simulink model "foc_7"  (R2024a)
settings: Solver=FixedStepAuto  StartTime=0.0  StopTime=3  FixedStep=1e-6  MaxStep=1e-5  RelTol=1e-3
undefined symbols (not defined in the file): DiscIntNeverNeededParam, Ki, Ki_s, Kp, Kp_s, L, lambda, ma, p, R, T_period, Vdc
libraries: simulink x13, spsIGBTDiodeLib x6, spsSeriesRLCBranchLib x6, eeGeneralControl x6, spsCurrentMeasurementLib x3, spsPermanentMagnetSynchronousMachineLib x2, spsDCVoltageSourceLib x1, spsStairGeneratorLib x1, spspowerguiLib x1
(part 1 of 2)
settings Model: Creator=Abdo  LastModifiedBy=kareem
settings SolverCC: ZeroCrossAlgorithm=Adaptive  AlgebraicLoopSolver=TrustRegion
settings OptimizationCC: DefaultParameterBehavior=Inlined  EnhancedBackFolding=on  PassReuseOutputArgsAs=Individual arguments  ZeroExternalMemoryAtStartup=off  ZeroInternalMemoryAtStartup=off  OptimizeBlockOrder=speed  DifferentSizesBufferReuse=on  OptimizationCustomize=off  EfficientTunableParamExpr=on
settings DebuggingCC: IgnoredZcDiagnostic=none  ParameterTunabilityLossMsg=error  ArithmeticOperatorsInVariantConditions=warning
settings HardwareCC: ProdBitPerChar=16  ProdBitPerInt=16  ProdBitPerPointer=32  ProdBitPerSizeT=32  ProdBitPerPtrDiffT=32  ProdLargestAtomicInteger=Integer  ProdLargestAtomicFloat=None  ProdWordSize=16  ProdHWDeviceType=Texas Instruments->C2000
settings SFSimCC: MATLABDynamicMemAlloc=off  CustomCodeUndefinedFunction=UseInterfaceOnly
settings RTWCC: Description=Embedded Coder  SystemTargetFile=ert.tlc  TemplateMakefile=ert_default_tmf  PortableWordSizes=on  GPUComputeCapability=3.5
settings CodeAppCC: ForceParamTrailComments=on  IgnoreCustomStorageClasses=off  OperatorAnnotations=on  SimulinkDataObjDesc=on  SFDataObjDesc=on  InsertBlockDesc=on
settings ERTTargetCC: TargetLangStandard=C99 (ISO)  GenerateSampleERTMain=on  InlinedParameterPlacement=NonHierarchical  ERTCustomFileTemplate=example_file_process.tlc

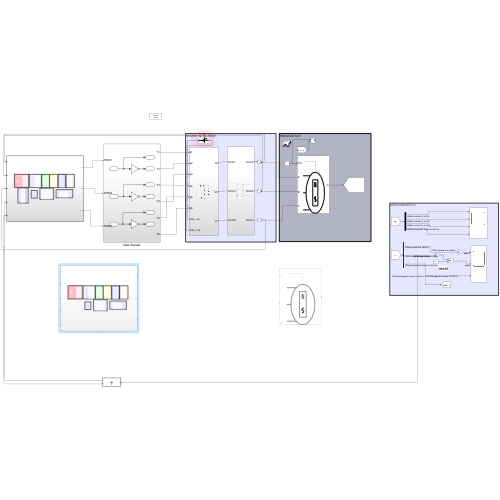
[thumbnail: Simulink's stored preview of the top-level diagram]
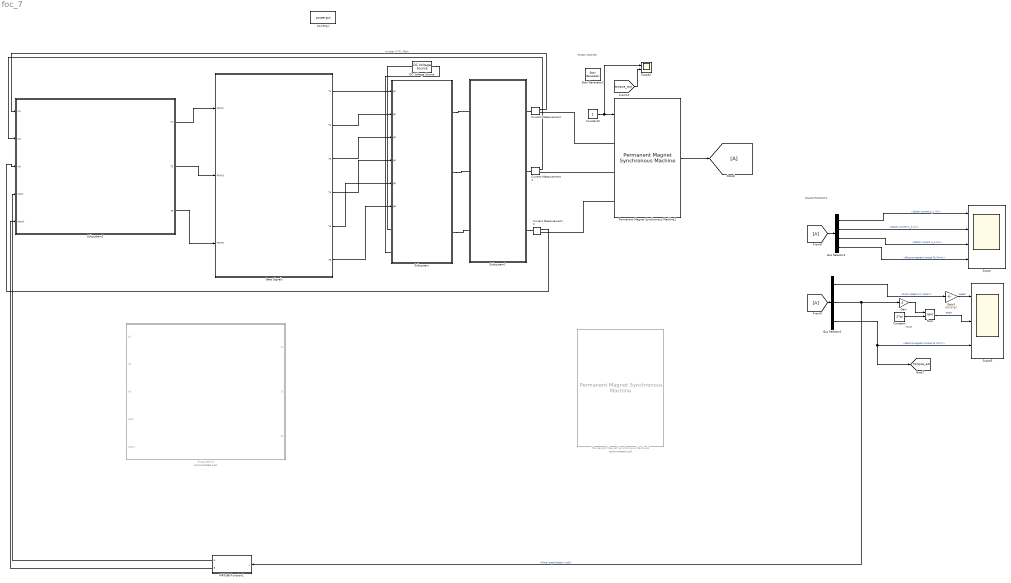
== system foc_7 ==
  note: MEASUREMENTS
  note: PMSM MOTOR
  note: inveter & RL filter
  note: reset
  Bus Selector1 : BusSelector  OutputSignals=Stator current is_c (A),Stator current is_b (A),Stator current is_a (A),Electromagnetic torque Te (N*m)
  Bus Selector2 : BusSelector  OutputSignals=Rotor speed wm (rad/s),Rotor angle thetam (rad),Electromagnetic torque Te (N*m)
  Constant : Constant  Value=2*pi
  Constant3 : Constant
  Current Measurement : spsCurrentMeasurementLib/Current Measurement  PhasorSimulation=off  OutputType=Complex  PSBequivalent=0
  Current Measurement1 : spsCurrentMeasurementLib/Current Measurement  PhasorSimulation=off  OutputType=Complex  PSBequivalent=0
  Current Measurement2 : spsCurrentMeasurementLib/Current Measurement  PhasorSimulation=off  OutputType=Complex  PSBequivalent=0
  DC Voltage Source : spsDCVoltageSourceLib/DC Voltage Source  Amplitude=Vdc  Measurements=None
  From8 : From
  From9 : From
  Gain : Gain  Gain=4
  Gain3 : Gain  Gain=60/(2*pi)
  Gate Signals : Subsystem
  Goto8 : Goto
  MATLAB Function1 : MATLAB Function  TreatAsAtomicUnit=on
  Permanent Magnet Synchronous Machine1 : spsPermanentMagnetSynchronousMachineLib/Permanent Magnet Synchronous Machine  NbPhases=3  FluxDistribution=Sinusoidal  RotorType=Round  MechanicalLoad=Torque Tm  PresetModel=No  ShowDetailedParameters=on  MeasurementBus=off  Resistance=2.9  Inductance=8.5e-3  dqInductances=[8.5e-3,8.5e-3]  La=0.0124  MachineConstant=Flux linkage established by magnets (V.s)  Flux=0.37/3  VoltageCst=89.4808  TorqueCst=0.74  Flat=120  Mechanical=[0.000026 0.000955 4 0.03]  PolePairs=4  InitialConditions=[0,0, 0,0]  InitialConditions5ph=[0 0 0 0 0 0]  RefAngle=Aligned with phase A axis (original Park)  IterativeDiscreteModel=Backward Euler robust  TsBlock=-1  TsPowergui=0
  Permanent Magnet Synchronous Machine3 : spsPermanentMagnetSynchronousMachineLib/Permanent Magnet Synchronous Machine  Commented=on  NbPhases=3  FluxDistribution=Sinusoidal  RotorType=Round  MechanicalLoad=Torque Tm  PresetModel=No  ShowDetailedParameters=on  MeasurementBus=off  Resistance=R  Inductance=8.5e-3  dqInductances=[8.5e-3,8.5e-3]  La=L  MachineConstant=Flux linkage established by magnets (V.s)  Flux=lambda  VoltageCst=62.5906  TorqueCst=0.51762  Flat=120  Mechanical=[0.000026 0.000955 4 0.03]  PolePairs=8  InitialConditions=[0 0 0 0]  InitialConditions5ph=[0 0 0 0 0 0]  RefAngle=Aligned with phase A axis (original Park)  IterativeDiscreteModel=Backward Euler robust  TsBlock=-1  TsPowergui=0
  Rem : Math  Operator=rem  SignedPower=on
  Scope : Scope  NumInputPorts=4
  Scope2 : Scope  NumInputPorts=2
  Scope5 : Scope  NumInputPorts=3
  Stair Generator2 : spsStairGeneratorLib/Stair Generator  t=[0 0.15 0.3 0.5 0.75 1 2 2.5]  e=[0 0.5 1 2 2.7 0.5 4 6]  Ts=0
  Subsystem : Subsystem
  Subsystem1 : Subsystem
  Subsystem2 : Subsystem  TreatAsAtomicUnit=on
  Subsystem3 : Subsystem  Commented=on  TreatAsAtomicUnit=on
  powergui : spspowerguiLib/powergui  Priority=1  SimulationMode=Discrete  SampleTime=1e-6  frequency=60  Iterations=50  frequencyindice=0  Pbase=100e6  ErrMax=1e-4  UnitsV=kV  UnitsW=MW  buscounter=0  FunctionMessages=off  echomessages=off  EnableUseOfTLC=off  CurrentSourceSwitches=off  DisableSnubberDevices=off  DisableRonSwitches=off  DisableVfSwitches=off  DisplayEquations=off  AutomaticDiscreteSolvers=off  SolverType=Tustin/Backward Euler (TBE)  Interpol=off  ExternalGateDelay=off  methode=off  Ts=100  x0status=blocks  SPID=on  SwTol=0  HookPort=off  NonlinearTolerance=1e-4  nMaxIteration=100  ContinueOnMaxIteration=off  RestoreLinks=warning  ResistiveCurrentMeasurement=off  Frange=[0:2:500]  Ylog=off  Xlog=on  ShowGrid=off  save=off  variable=ZData  structure=0  ZoomFFT=off  StartTime=0.0  cycles=1  DisplayStyle=1  fundamental=60  FreqAxis=off  MaxFrequency=1000  frequencyindicesteady=1  RmsSteady=1  display=off
  tag scope: torque_act=global
  wires:
  Gain/1 -> Rem/1
  Current Measurement2/1 -> Subsystem2/3(In3)
  Current Measurement1/1 -> Subsystem2/2(In2)
  Current Measurement/1 -> Subsystem2/1(In1)
  Bus Selector2/2 -> MATLAB Function1/1(u), Gain/1  "<Rotor angle thetam (rad)>"
  Constant/1 -> Rem/2
  Rem/1 -> Scope5/2  "angle"
  Permanent Magnet Synchronous Machine1/1 -> Goto8/1
  Bus Selector2/1 -> Gain3/1  "<Rotor speed wm (rad/s)>"
  Bus Selector1/1 -> Scope/1  "<Stator current is_c (A)>"
  Bus Selector1/2 -> Scope/2  "<Stator current is_b (A)>"
  Bus Selector1/3 -> Scope/3  "<Stator current is_a (A)>"
  Bus Selector1/4 -> Scope/4  "<Electromagnetic torque Te (N*m)>"
  Gain3/1 -> Scope5/1  "speed"
  Bus Selector2/3 -> [torque_act], Scope5/3  "<Electromagnetic torque Te (N*m)>"
  From8/1 -> Bus Selector1/1
  From9/1 -> Bus Selector2/1
  Constant3/1 -> Permanent Magnet Synchronous Machine1/1, Scope2/1
  [torque_act] -> Scope2/2
  MATLAB Function1/1(A) -> Subsystem2/4(Input)
  MATLAB Function1/2(B) -> Subsystem2/5(Input1)
  Gate Signals/1(T1) -> Subsystem/1(g1)
  Gate Signals/2(T2) -> Subsystem/2(g2)
  Gate Signals/3(T3) -> Subsystem/3(g3)
  Gate Signals/4(T4) -> Subsystem/4(g4)
  Gate Signals/5(T5) -> Subsystem/5(g5)
  Gate Signals/6(T6) -> Subsystem/6(g6)
  Subsystem2/1(T1) -> Gate Signals/1(PWM1)
  Subsystem2/2(T3) -> Gate Signals/2(PWM3)
  Subsystem2/3(T5) -> Gate Signals/3(PWM5)
  connections:
  Permanent Magnet Synchronous Machine1/LConn1 -- Current Measurement/RConn1
  Subsystem/LConn1 -- DC Voltage Source/LConn1
  Permanent Magnet Synchronous Machine1/LConn2 -- Current Measurement1/RConn1
  DC Voltage Source/RConn1 -- Subsystem/LConn2
  Permanent Magnet Synchronous Machine1/LConn3 -- Current Measurement2/RConn1
  Subsystem/RConn1 -- Subsystem1/LConn1
  Subsystem1/RConn1 -- Current Measurement/LConn1
  Subsystem/RConn2 -- Subsystem1/LConn2
  Subsystem1/RConn2 -- Current Measurement1/LConn1
  Subsystem1/RConn3 -- Current Measurement2/LConn1
  Subsystem/RConn3 -- Subsystem1/LConn3

== system foc_7/Gate Signals ==
  PWM1 : Inport
  PWM3 : Inport  Port=2
  PWM5 : Inport  Port=3
  NOT : Logic  Operator=NOT  IconShape=distinctive  AllPortsSameDT=off  OutDataTypeStr=boolean
  NOT1 : Logic  Operator=NOT  IconShape=distinctive  AllPortsSameDT=off  OutDataTypeStr=boolean
  NOT2 : Logic  Operator=NOT  IconShape=distinctive  AllPortsSameDT=off  OutDataTypeStr=boolean
  T1 : Outport
  T2 : Outport  Port=2
  T3 : Outport  Port=3
  T4 : Outport  Port=4
  T5 : Outport  Port=5
  T6 : Outport  Port=6
  wires:
  PWM1/1 -> T1/1, NOT/1
  NOT/1 -> T4/1
  NOT1/1 -> T6/1
  PWM3/1 -> T3/1, NOT1/1
  PWM5/1 -> T5/1, NOT2/1
  NOT2/1 -> T2/1

== system foc_7/Subsystem ==
  g1 : Inport
  g2 : Inport  Port=2
  g3 : Inport  Port=3
  g4 : Inport  Port=4
  g5 : Inport  Port=5
  g6 : Inport  Port=6
  IGBT/Diode{,1..5} (6 alike) : spsIGBTDiodeLib/IGBT//Diode  Ron=1e-3  Rs=1e5  Cs=inf  Measurements=off
  Vdc_-ve : PMIOPort  Side=Left
  Vdc_+ve : PMIOPort  Port=2  Side=Left
  Va : PMIOPort  Port=3  Side=Right
  Vb : PMIOPort  Port=4  Side=Right
  Vc : PMIOPort  Port=5  Side=Right
  wires:
  g2/1 -> IGBT/Diode5/1
  g5/1 -> IGBT/Diode4/1
  g3/1 -> IGBT/Diode2/1
  g4/1 -> IGBT/Diode1/1
  g1/1 -> IGBT/Diode/1
  g6/1 -> IGBT/Diode3/1
  connections:
  IGBT/Diode5/LConn1 -- Vc/RConn1 -- IGBT/Diode4/RConn1
  Vb/RConn1 -- IGBT/Diode3/LConn1 -- IGBT/Diode2/RConn1
  IGBT/Diode5/RConn1 -- Vdc_-ve/RConn1 -- IGBT/Diode1/RConn1 -- IGBT/Diode3/RConn1
  IGBT/Diode4/LConn1 -- IGBT/Diode/LConn1 -- Vdc_+ve/RConn1 -- IGBT/Diode2/LConn1
  Va/RConn1 -- IGBT/Diode/RConn1 -- IGBT/Diode1/LConn1

== system foc_7/Subsystem1 ==
  Series RLC Branch10 : spsSeriesRLCBranchLib/Series RLC Branch  LConnTagsString=__new0  RConnTagsString=__new0  BranchType=R  Resistance=10e4  Inductance=1e-2  SetiL0=off  InitialCurrent=0  Capacitance=1e-6  Setx0=off  InitialVoltage=0  Measurements=None
  Series RLC Branch11 : spsSeriesRLCBranchLib/Series RLC Branch  LConnTagsString=__new0  RConnTagsString=__new0  BranchType=R  Resistance=10e4  Inductance=1e-2  SetiL0=off  InitialCurrent=0  Capacitance=1e-6  Setx0=off  InitialVoltage=0  Measurements=None
  Series RLC Branch6 : spsSeriesRLCBranchLib/Series RLC Branch  LConnTagsString=__new0  RConnTagsString=__new0  BranchType=L  Resistance=1  Inductance=4e-3  SetiL0=on  InitialCurrent=0  Capacitance=1e-6  Setx0=off  InitialVoltage=0  Measurements=None
  Series RLC Branch7 : spsSeriesRLCBranchLib/Series RLC Branch  LConnTagsString=__new0  RConnTagsString=__new0  BranchType=L  Resistance=1  Inductance=4e-3  SetiL0=on  InitialCurrent=0  Capacitance=1e-6  Setx0=off  InitialVoltage=0  Measurements=None
  Series RLC Branch8 : spsSeriesRLCBranchLib/Series RLC Branch  LConnTagsString=__new0  RConnTagsString=__new0  BranchType=L  Resistance=1  Inductance=4e-3  SetiL0=on  InitialCurrent=0  Capacitance=1e-6  Setx0=off  InitialVoltage=0  Measurements=None
  Series RLC Branch9 : spsSeriesRLCBranchLib/Series RLC Branch  LConnTagsString=__new0  RConnTagsString=__new0  BranchType=R  Resistance=10e4  Inductance=1e-2  SetiL0=off  InitialCurrent=0  Capacitance=1e-6  Setx0=off  InitialVoltage=0  Measurements=None
  Conn1 : PMIOPort  Side=Left
  Conn2 : PMIOPort  Port=2  Side=Right
  Conn3 : PMIOPort  Port=3  Side=Left
  Conn4 : PMIOPort  Port=4  Side=Right
  Conn5 : PMIOPort  Port=5  Side=Right
  Conn6 : PMIOPort  Port=6  Side=Left
  connections:
  Series RLC Branch8/LConn1 -- Series RLC Branch9/LConn1 -- Conn6/RConn1
  Series RLC Branch7/LConn1 -- Conn3/RConn1 -- Series RLC Branch10/LConn1
  Series RLC Branch7/RConn1 -- Conn4/RConn1 -- Series RLC Branch10/RConn1
  Series RLC Branch6/LConn1 -- Conn1/RConn1 -- Series RLC Branch11/LConn1
  Series RLC Branch6/RConn1 -- Conn2/RConn1 -- Series RLC Branch11/RConn1
  Series RLC Branch8/RConn1 -- Conn5/RConn1 -- Series RLC Branch9/RConn1

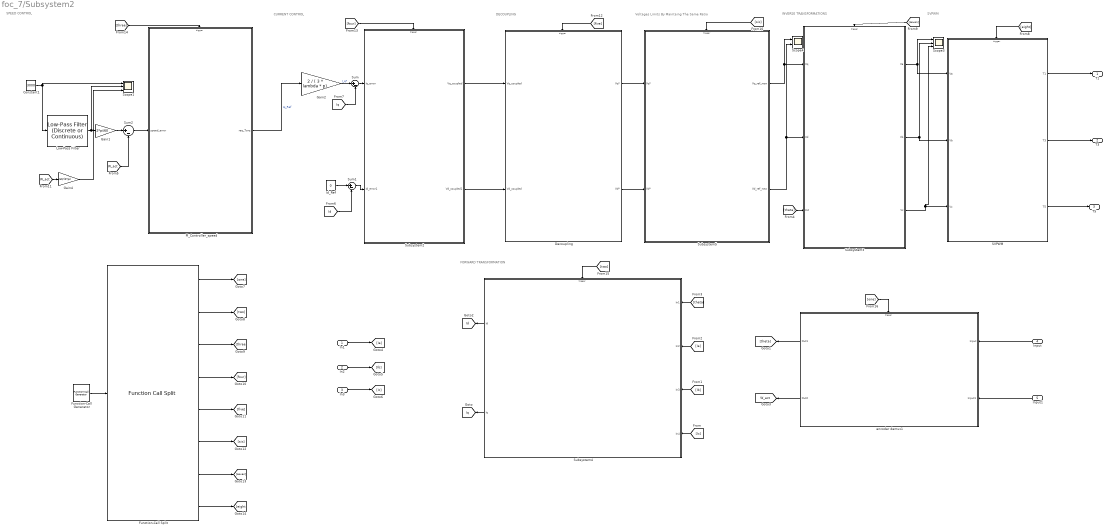
== system foc_7/Subsystem2 ==
  note: Voltages Limits By Maintaing The Same Ratio
  note: FORWARD TRANSFORMATION
  note: SPEED CONTROL
  note: CURRENT CONTROL
  note: DECOUPLING
  note: INVERSE TRANSFORMATIONS
  note: SVPWM
  In1 : Inport
  In2 : Inport  Port=2
  In3 : Inport  Port=3
  Input : Inport  Port=4
  Input1 : Inport  Port=5
  Constant1 : Constant  Value=3000
  Decoupling : Subsystem
  Function-Call Generator : simulink/Ports & Subsystems/Function-Call Generator  sample_time=1  numberOfIterations=1  DisallowWideOutput=off
  Function-Call Split : FunctionCallSplit  IconShape=distinctive  NumOutputPorts=8  OutputPortLayout=default
  Gain1 : Gain  Gain=2*pi/60
  Gain2 : Gain  Gain=2 / ( 3 * lambda * p)
  Gain4 : Gain  Gain=60/(2*pi)
  Id_Ref : Constant  Value=0
  "Low-Pass Filter " : eeGeneralControl/Low-Pass Filter (Discrete or Continuous)  K=1  T=1/100  B=inf  A=-inf  init_option=Inherited from block input  x0=0  Ts=-1
  PI_Controller_speed : Subsystem
  SVPWM : Subsystem
  Scope1 : Scope  NumInputPorts=3
  Scope3 : Scope  NumInputPorts=3
  Scope4 : Scope  NumInputPorts=2
  Subsystem2 : Subsystem
  Subsystem3 : Subsystem
  Subsystem4 : Subsystem
  Subsystem5 : Subsystem
  Sum : Sum  Inputs=|+-
  Sum1 : Sum  Inputs=|+-
  Sum2 : Sum  Inputs=|+-
  encoder demux1 : Subsystem
  T1 : Outport
  T3 : Outport  Port=2
  T5 : Outport  Port=3
  tag scope: Id=global, Iq=global, W_act=global
  wires:
  Gain4/1 -> Scope1/3
  Sum/1 -> Subsystem2/1(Iq_error)
  Constant1/1 -> "Low-Pass Filter "/1, Scope1/1
  Subsystem2/2(Vd_coupled1) -> Decoupling/2(Vd_coupled)
  Gain1/1 -> Sum2/1
  [Id] -> Sum1/2
  Decoupling/1(Vq*) -> Subsystem5/1(Vq*)
  Decoupling/2(Vd*) -> Subsystem5/2(Vd*)
  "Low-Pass Filter "/1 -> Scope1/2, Gain1/1
  Subsystem3/2(Vb) -> Scope3/2, SVPWM/2(Vb)
  Subsystem4/2(Iq) -> [Iq]
  Sum1/1 -> Subsystem2/2(Id_error1)
  Subsystem2/1(Vq_coupled) -> Decoupling/1(Vq_coupled)
  PI_Controller_speed/1(req_Torq) -> Gain2/1  "Iq_Ref"
  Subsystem5/2(Vd_ref_new) -> Subsystem3/2(Vd), Scope4/2
  Gain2/1 -> Sum/1  "I_q*"
  [W_act] -> Gain4/1
  Subsystem4/1(Id) -> [Id]
  Subsystem3/3(Vc) -> Scope3/3, SVPWM/3(Vc)
  Subsystem3/1(Va) -> Scope3/1, SVPWM/1(Va)
  Subsystem5/1(Vq_ref_new) -> Scope4/1, Subsystem3/1(Vq)
  Id_Ref/1 -> Sum1/1
  [Ic] -> Subsystem4/4(In4)
  [W_act] -> Sum2/2
  SVPWM/1(T1) -> T1/1
  [Iq] -> Sum/2
  Sum2/1 -> PI_Controller_speed/1(speed_error)
  [Ib] -> Subsystem4/3(In3)
  [theta] -> Subsystem4/1(In1)
  [Ia] -> Subsystem4/2(In2)
  [theta] -> Subsystem3/3(In2)
  SVPWM/3(T5) -> T5/1
  SVPWM/2(T3) -> T3/1
  Input/1 -> encoder demux1/1(Input)
  Input1/1 -> encoder demux1/2(Input1)
  encoder demux1/1(Out1) -> [theta]
  encoder demux1/2(Out2) -> [W_act]
  In1/1 -> [Ia]
  In2/1 -> [Ib]
  In3/1 -> [Ic]
  Function-Call Generator/1 -> Function-Call Split/1
  Function-Call Split/8 -> [eight]
  Function-Call Split/7 -> [seven]
  Function-Call Split/6 -> [six]
  Function-Call Split/5 -> [five]
  Function-Call Split/4 -> [four]
  Function-Call Split/3 -> [three]
  Function-Call Split/2 -> [two]
  Function-Call Split/1 -> [one]
  [one] -> encoder demux1/Trigger
  [two] -> Subsystem4/Trigger
  [three] -> PI_Controller_speed/Trigger
  [four] -> Subsystem2/Trigger
  [five] -> Decoupling/Trigger
  [eight] -> SVPWM/Trigger
  [seven] -> Subsystem3/Trigger
  [six] -> Subsystem5/Trigger

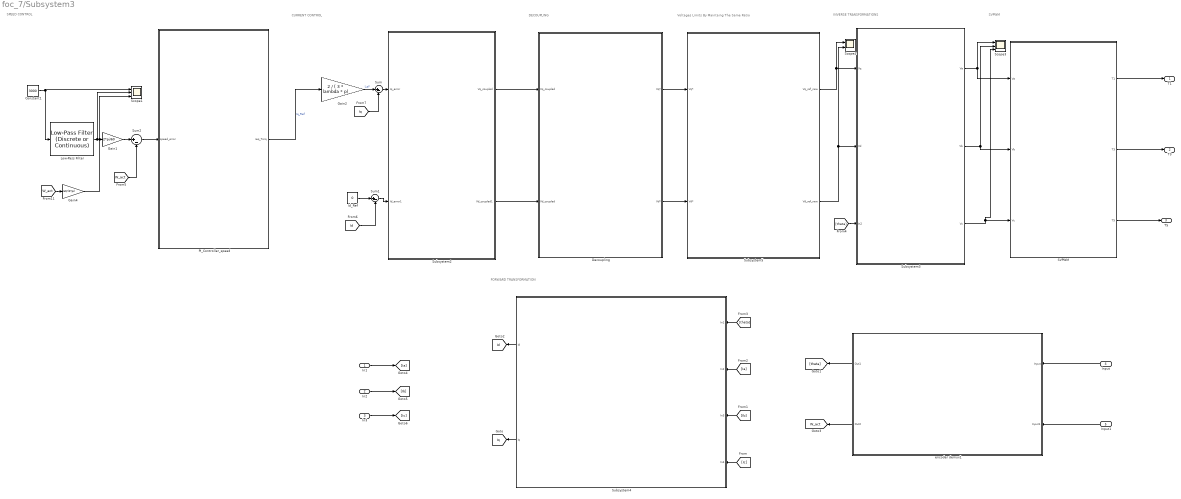
== system foc_7/Subsystem3 ==
  note: Voltages Limits By Maintaing The Same Ratio
  note: FORWARD TRANSFORMATION
  note: SPEED CONTROL
  note: CURRENT CONTROL
  note: DECOUPLING
  note: INVERSE TRANSFORMATIONS
  note: SVPWM
  In1 : Inport
  In2 : Inport  Port=2
  In3 : Inport  Port=3
  Input : Inport  Port=4
  Input1 : Inport  Port=5
  Constant1 : Constant  Value=3000
  Decoupling : Subsystem
  Gain1 : Gain  Gain=2*pi/60
  Gain2 : Gain  Gain=2 / ( 3 * lambda * p)
  Gain4 : Gain  Gain=60/(2*pi)
  Id_Ref : Constant  Value=0
  "Low-Pass Filter " : eeGeneralControl/Low-Pass Filter (Discrete or Continuous)  K=1  T=1/100  B=inf  A=-inf  init_option=Inherited from block input  x0=0  Ts=-1
  PI_Controller_speed : Subsystem
  SVPWM : Subsystem
  Scope1 : Scope  NumInputPorts=3
  Scope3 : Scope  NumInputPorts=3
  Scope4 : Scope  NumInputPorts=2
  Subsystem2 : Subsystem
  Subsystem3 : Subsystem
  Subsystem4 : Subsystem
  Subsystem5 : Subsystem
  Sum : Sum  Inputs=|+-
  Sum1 : Sum  Inputs=|+-
  Sum2 : Sum  Inputs=|+-
  encoder demux1 : Subsystem
  T1 : Outport
  T3 : Outport  Port=2
  T5 : Outport  Port=3
  tag scope: Id=global, Iq=global, W_act=global
  wires:
  Gain4/1 -> Scope1/3
  Sum/1 -> Subsystem2/1(Iq_error)
  Constant1/1 -> "Low-Pass Filter "/1, Scope1/1
  Subsystem2/2(Vd_coupled1) -> Decoupling/2(Vd_coupled)
  Gain1/1 -> Sum2/1
  [Id] -> Sum1/2
  Decoupling/1(Vq*) -> Subsystem5/1(Vq*)
  Decoupling/2(Vd*) -> Subsystem5/2(Vd*)
  "Low-Pass Filter "/1 -> Scope1/2, Gain1/1
  Subsystem3/2(Vb) -> SVPWM/2(Vb), Scope3/2
  Subsystem4/2(Iq) -> [Iq]
  Sum1/1 -> Subsystem2/2(Id_error1)
  Subsystem2/1(Vq_coupled) -> Decoupling/1(Vq_coupled)
  PI_Controller_speed/1(req_Torq) -> Gain2/1  "Iq_Ref"
  Subsystem5/2(Vd_ref_new) -> Subsystem3/2(Vd), Scope4/2
  Gain2/1 -> Sum/1  "I_q*"
  [W_act] -> Gain4/1
  Subsystem4/1(Id) -> [Id]
  Subsystem3/3(Vc) -> Scope3/3, SVPWM/3(Vc)
  Subsystem3/1(Va) -> Scope3/1, SVPWM/1(Va)
  Subsystem5/1(Vq_ref_new) -> Scope4/1, Subsystem3/1(Vq)
  Id_Ref/1 -> Sum1/1
  [Ic] -> Subsystem4/4(In4)
  [W_act] -> Sum2/2
  SVPWM/1(T1) -> T1/1
  [Iq] -> Sum/2
  Sum2/1 -> PI_Controller_speed/1(speed_error)
  [Ib] -> Subsystem4/3(In3)
  [theta] -> Subsystem4/1(In1)
  [Ia] -> Subsystem4/2(In2)
  [theta] -> Subsystem3/3(In2)
  SVPWM/3(T5) -> T5/1
  SVPWM/2(T3) -> T3/1
  Input/1 -> encoder demux1/1(Input)
  Input1/1 -> encoder demux1/2(Input1)
  encoder demux1/1(Out1) -> [theta]
  encoder demux1/2(Out2) -> [W_act]
  In1/1 -> [Ia]
  In2/1 -> [Ib]
  In3/1 -> [Ic]

== system foc_7/Subsystem2/Decoupling ==
  Vq_coupled : Inport
  Vd_coupled : Inport  Port=2
  Trigger : TriggerPort  TriggerType=function-call  VariantControl=Variant  PortDimensions=1
  Add : Sum  Inputs=+++
  Add1 : Sum  Inputs=+-
  Constant1 : Constant  Value=lambda
  Constant2 : Constant  Value=L
  Constant3 : Constant  Value=L
  Product : Product
  Product1 : Product  Inputs=3
  Product2 : Product  Inputs=3
  Vq* : Outport
  Vd* : Outport  Port=2
  wires:
  [W_act] -> Product1/1
  Product/1 -> Add/1
  Product1/1 -> Add/2
  [W_act] -> Product2/1
  Product2/1 -> Add1/2
  Constant3/1 -> Product2/3
  Constant2/1 -> Product1/3
  Constant1/1 -> Product/2
  [Id] -> Product2/2
  [W_act] -> Product/1
  [Iq] -> Product1/2
  Vd_coupled/1 -> Add1/1
  Add1/1 -> Vd*/1  "Vd"
  Add/1 -> Vq*/1  "Vq"
  Vq_coupled/1 -> Add/3

== system foc_7/Subsystem2/PI_Controller_speed ==
  speed_error : Inport
  Trigger : TriggerPort  TriggerType=function-call  VariantControl=Variant  PortDimensions=1
  Abs : Abs  SaturateOnIntegerOverflow=off
  Add : Sum
  Add1 : Sum  Inputs=+-
  Compare To Constant1 : simulink/Logic and Bit Operations/Compare To Constant  relop=<=  const=1e-4  OutDataTypeStr=boolean
  Gain3 : Gain  Gain=Kp_s
  Gain4 : Gain  Gain=Ki_s
  Integrator (Discrete or Continuous) : eeGeneralControl/Integrator (Discrete or Continuous)  LabelModeActiveChoice=Discrete  ExternalReset=level  LimitType=Anti-windup  B=4  A=-inf  Ts=-1
  Product : Product
  Saturation : Saturate  UpperLimit=3.8  LowerLimit=-3.8
  req_Torq : Outport
  wires:
  Saturation/1 -> Add1/2, req_Torq/1
  Add/1 -> Add1/1, Saturation/1
  Gain3/1 -> Add/1
  Integrator (Discrete or Continuous)/1 -> Add/2
  Gain4/1 -> Product/1
  Add1/1 -> Abs/1
  Abs/1 -> Compare To Constant1/1
  speed_error/1 -> Gain3/1, Gain4/1
  Product/1 -> Integrator (Discrete or Continuous)/1
  Compare To Constant1/1 -> Product/2

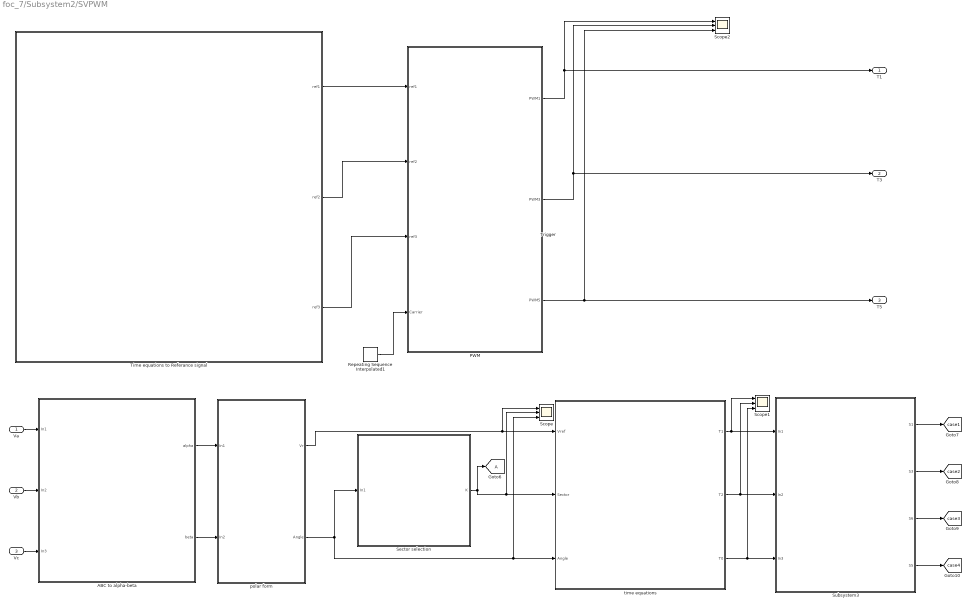
== system foc_7/Subsystem2/SVPWM ==
  Va : Inport
  Vb : Inport  Port=2
  Vc : Inport  Port=3
  Trigger : TriggerPort  TriggerType=function-call  VariantControl=Variant  PortDimensions=1
  ABC to alpha-beta : Subsystem
  Goto6 : Goto  TagVisibility=global
  PWM : Subsystem
  Repeating Sequence Interpolated1 : simulink/Sources/Repeating Sequence Interpolated  OutValues="[ 0 1/15000  1e-6  ]"  TimeValues=[ 0 1/40000 1/20001]  LookUpMeth=Interpolation-Use End Values  tsamp=1e-6  OutMin=[]  OutMax=[]  OutDataTypeStr=double  OutputDataTypeScalingMode=double  OutDataType=fixdt(0,8)  OutScaling=2^-10
  Scope : Scope  NumInputPorts=3
  Scope1 : Scope  NumInputPorts=3
  Scope2 : Scope  NumInputPorts=3
  Sector selection : Subsystem
  Subsystem3 : Subsystem
  Time equations to Referance signal : Subsystem
  polar form : Subsystem
  time equations : Subsystem
  T1 : Outport
  T3 : Outport  Port=2
  T5 : Outport  Port=3
  tag scope: case1=global, case2=global, case3=global, case4=global
  wires:
  Vb/1 -> ABC to alpha-beta/2(In2)
  time equations/1(T1) -> Scope1/1, Subsystem3/1(In1)
  Va/1 -> ABC to alpha-beta/1(In1)
  Time equations to Referance signal/1(ref1) -> PWM/1(ref1)
  Time equations to Referance signal/2("ref2 ") -> PWM/2(ref2)
  Time equations to Referance signal/3(ref3) -> PWM/3(ref3)
  Vc/1 -> ABC to alpha-beta/3(In3)
  ABC to alpha-beta/1(alpha) -> polar form/1(In1)
  ABC to alpha-beta/2(beta) -> polar form/2(In2)
  PWM/1(PWM1) -> T1/1, Scope2/1
  PWM/2(PWM3) -> T3/1, Scope2/2
  PWM/3(PWM5) -> T5/1, Scope2/3
  polar form/2(Angle) -> Sector selection/1(In1), time equations/3(Angle), Scope/3
  polar form/1(Vr) -> Scope/1, time equations/1(Vref)
  Sector selection/1(K) -> Scope/2, time equations/2(Sector), Goto6/1
  Subsystem3/2(S3) -> [case2]
  Subsystem3/1(S1) -> [case1]
  time equations/3(T0) -> Subsystem3/3(In3), Scope1/3
  time equations/2(T2) -> Scope1/2, Subsystem3/2(In2)
  Subsystem3/4(S5) -> [case4]
  Subsystem3/3(S6) -> [case3]
  Repeating Sequence Interpolated1/1 -> PWM/4(Carrier)

== system foc_7/Subsystem2/Subsystem2 ==
  Iq_error : Inport
  Id_error1 : Inport  Port=2
  Trigger : TriggerPort  TriggerType=function-call  VariantControl=Variant  PortDimensions=1
  PI_Controller_Id : Subsystem
  PI_Controller_Iq : Subsystem
  Vq_coupled : Outport
  Vd_coupled1 : Outport  Port=2
  wires:
  PI_Controller_Id/1(Vd_coupled) -> Vd_coupled1/1
  Id_error1/1 -> PI_Controller_Id/1(Id_error)
  Iq_error/1 -> PI_Controller_Iq/1(Iq_error)
  PI_Controller_Iq/1(Vq_coupled) -> Vq_coupled/1

== system foc_7/Subsystem2/Subsystem3 ==
  Vq : Inport
  Vd : Inport  Port=2
  In2 : Inport  Port=3
  Trigger : TriggerPort  TriggerType=function-call  VariantControl=Variant  PortDimensions=1
  Add : Sum
  Add1 : Sum  Inputs=-+
  Add2 : Sum  Inputs=--
  Add3 : Sum  Inputs=+-
  Cosine : Trigonometry  Operator=cos
  Cosine1 : Trigonometry
  Gain : Gain  Gain=sqrt(3)
  Gain1 : Gain  Gain=1/2
  Gain2 : Gain  Gain=1/2
  Product{,1..3} (4 alike) : Product
  Sin : Trigonometry
  Sin1 : Trigonometry  Operator=cos
  Va : Outport
  Vb : Outport  Port=2
  Vc : Outport  Port=3
  wires:
  Add/1 -> Add3/2, Add2/2, Va/1  "V_beta"
  Product2/1 -> Add1/2
  Product3/1 -> Add1/1
  Cosine/1 -> Product/1
  Sin1/1 -> Product2/1
  Sin/1 -> Product1/1
  Product/1 -> Add/2
  Vd/1 -> Product1/2, Product2/2
  In2/1 -> Sin/1, Cosine/1, Cosine1/1, Sin1/1
  Product1/1 -> Add/1
  Cosine1/1 -> Product3/2
  Add1/1 -> Gain/1  "V_alpha"
  Vq/1 -> Product3/1, Product/2
  Gain1/1 -> Vc/1  "Vc"
  Add3/1 -> Gain2/1
  Gain/1 -> Add2/1, Add3/1
  Add2/1 -> Gain1/1
  Gain2/1 -> Vb/1  "Vb"

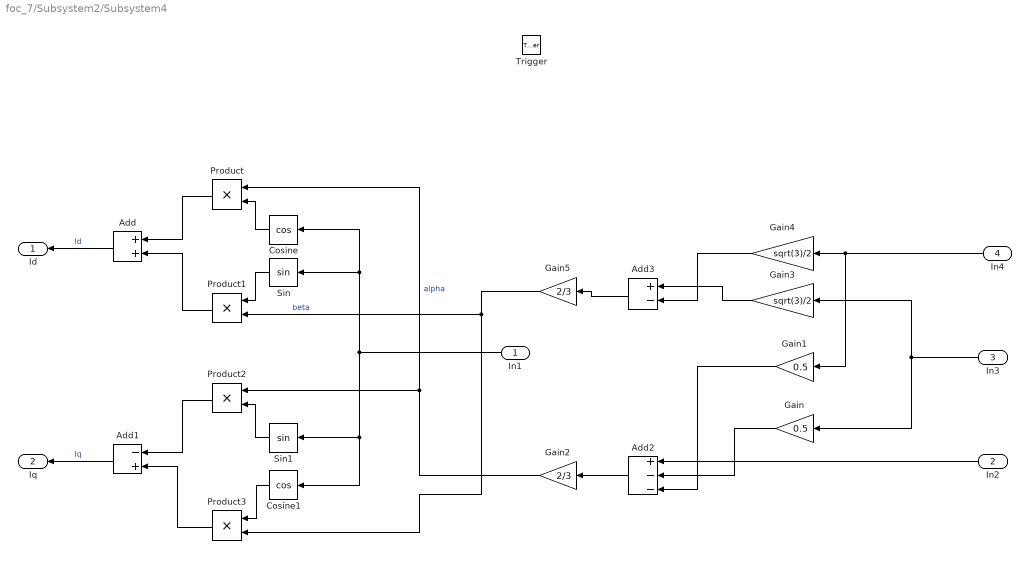
== system foc_7/Subsystem2/Subsystem4 ==
  In1 : Inport
  In2 : Inport  Port=2
  In3 : Inport  Port=3
  In4 : Inport  Port=4
  Trigger : TriggerPort  TriggerType=function-call  VariantControl=Variant  PortDimensions=1
  Add : Sum
  Add1 : Sum  Inputs=-+
  Add2 : Sum  Inputs=+--
  Add3 : Sum  Inputs=+-
  Cosine : Trigonometry  Operator=cos
  Cosine1 : Trigonometry  Operator=cos
  Gain : Gain  Gain=0.5
  Gain1 : Gain  Gain=0.5
  Gain2 : Gain  Gain=2/3
  Gain3 : Gain  Gain=sqrt(3)/2
  Gain4 : Gain  Gain=sqrt(3)/2
  Gain5 : Gain  Gain=2/3
  Product{,1..3} (4 alike) : Product
  Sin : Trigonometry
  Sin1 : Trigonometry
  Id : Outport
  Iq : Outport  Port=2
  wires:
  Add1/1 -> Iq/1  "Iq"
  Add/1 -> Id/1  "Id"
  Product3/1 -> Add1/2
  Product1/1 -> Add/2
  Sin1/1 -> Product2/2
  Sin/1 -> Product1/1
  Product/1 -> Add/1
  Cosine1/1 -> Product3/1
  In1/1 -> Cosine/1, Sin/1, Cosine1/1, Sin1/1
  Product2/1 -> Add1/1
  Cosine/1 -> Product/2
  Gain5/1 -> Product3/2, Product1/2  "beta"
  Gain2/1 -> Product/1, Product2/1  "alpha"
  Add2/1 -> Gain2/1
  In2/1 -> Add2/1
  Gain/1 -> Add2/2
  In4/1 -> Gain1/1, Gain4/1
  Gain1/1 -> Add2/3
  Add3/1 -> Gain5/1
  Gain4/1 -> Add3/2
  In3/1 -> Gain/1, Gain3/1
  Gain3/1 -> Add3/1

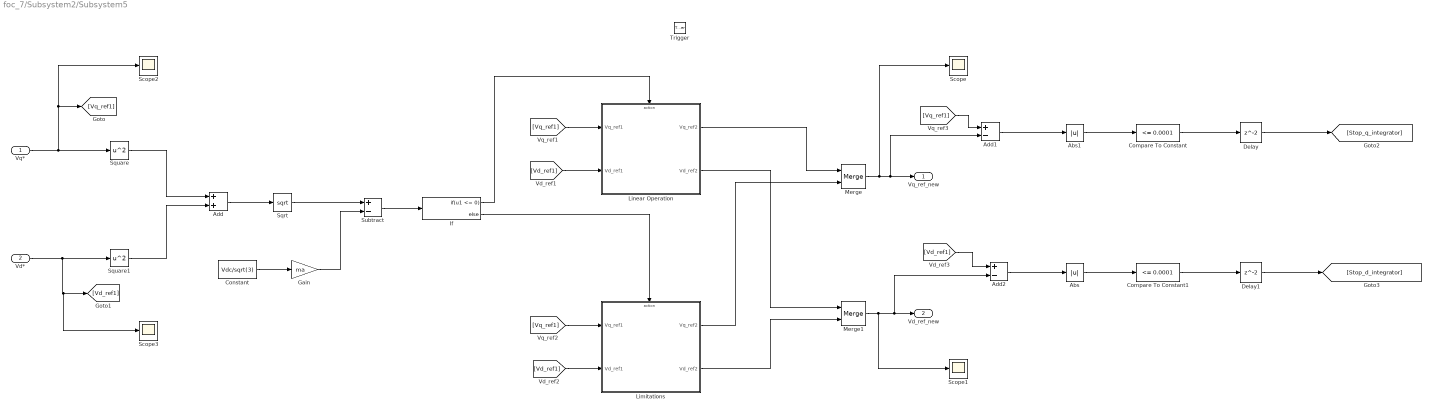
== system foc_7/Subsystem2/Subsystem5 ==
  Vq* : Inport
  Vd* : Inport  Port=2
  Trigger : TriggerPort  TriggerType=function-call  VariantControl=Variant  PortDimensions=1
  Abs : Abs  SaturateOnIntegerOverflow=off
  Abs1 : Abs  SaturateOnIntegerOverflow=off
  Add : Sum
  Add1 : Sum  Inputs=+-
  Add2 : Sum  Inputs=+-
  Compare To Constant : simulink/Logic and Bit Operations/Compare To Constant  relop=<=  const=0.0001  OutDataTypeStr=boolean
  Compare To Constant1 : simulink/Logic and Bit Operations/Compare To Constant  relop=<=  const=0.0001  OutDataTypeStr=boolean
  Constant : Constant  Value=Vdc/sqrt(3)
  Delay : Delay
  Delay1 : Delay
  Gain : Gain  Gain=ma
  If : If  IfExpression=u1 <= 0
  Limitations : Subsystem  TreatAsAtomicUnit=on
  "Linear Operation " : Subsystem  TreatAsAtomicUnit=on
  Merge : Merge
  Merge1 : Merge
  Scope{,1..3} (4 alike) : Scope
  Sqrt : Sqrt
  Square : Math  Operator=square  SignedPower=on
  Square1 : Math  Operator=square  SignedPower=on
  Subtract : Sum  Inputs=+-
  Vq_ref_new : Outport
  Vd_ref_new : Outport  Port=2
  wires:
  Vd*/1 -> Scope3/1, [Vd_ref1], Square1/1
  Vq*/1 -> Scope2/1, [Vq_ref1], Square/1
  Square/1 -> Add/1
  Square1/1 -> Add/2
  Add/1 -> Sqrt/1
  Constant/1 -> Gain/1
  Sqrt/1 -> Subtract/1
  Gain/1 -> Subtract/2
  Subtract/1 -> If/1
  [Vq_ref1] -> "Linear Operation "/1(Vq_ref1)
  [Vd_ref1] -> "Linear Operation "/2(Vd_ref1)
  If/1 -> "Linear Operation "/Action
  If/2 -> Limitations/Action
  [Vq_ref1] -> Limitations/1(Vq_ref1)
  [Vd_ref1] -> Limitations/2(Vd_ref1)
  Limitations/2(Vd_ref2) -> Merge1/2
  "Linear Operation "/2(Vd_ref2) -> Merge1/1
  Limitations/1(Vq_ref2) -> Merge/2
  "Linear Operation "/1(Vq_ref2) -> Merge/1
  Merge/1 -> Scope/1, Add1/2, Vq_ref_new/1
  Merge1/1 -> Scope1/1, Add2/2, Vd_ref_new/1
  [Vq_ref1] -> Add1/1
  [Vd_ref1] -> Add2/1
  Add2/1 -> Abs/1
  Add1/1 -> Abs1/1
  Abs1/1 -> Compare To Constant/1
  Abs/1 -> Compare To Constant1/1
  Compare To Constant/1 -> Delay/1
  Compare To Constant1/1 -> Delay1/1
  Delay/1 -> [Stop_q_integrator]
  Delay1/1 -> [Stop_d_integrator]

== system foc_7/Subsystem2/encoder demux1 ==
  Input : Inport
  Input1 : Inport  Port=2
  Trigger : TriggerPort  TriggerType=function-call  VariantControl=Variant  PortDimensions=1
  Add1 : Sum
  Constant2 : Constant
  Constant3 : Constant  Value=2*pi
  Constant4 : Constant  Value=0
  Data Type Conversion : DataTypeConversion  SaturateOnIntegerOverflow=off  RndMeth=Floor
  Data Type Conversion1 : DataTypeConversion  SaturateOnIntegerOverflow=off  RndMeth=Floor
  Detect Rise Positive : simulink/Logic and Bit Operations/Detect Rise Positive  vinit=0  OutDataTypeStr=uint8
  Discrete Derivative : simulink/Discrete/Discrete Derivative  gainval=1.0  ICPrevScaledInput=0.0  OutMin=[]  OutMax=[]  OutDataType=fixdt(1, 16)  OutScaling=2^-10  DoSatur=off
  Gain : Gain
  Gain1 : Gain  Gain=-1
  Gain2 : Gain  Gain=2*pi /2000
  Gain3 : Gain  Gain=4
  "Low-Pass Filter " : eeGeneralControl/Low-Pass Filter (Discrete or Continuous)  K=1  T=1/100  B=inf  A=-inf  init_option=Inherited from block input  x0=0  Ts=-1
  Rem : Math  Operator=rem
  Scope : Scope  NumInputPorts=3
  Switch : Switch  Criteria=u2 > Threshold  SaturateOnIntegerOverflow=off  InputSameDT=off
  Switch2 : Switch  Criteria=u2 > Threshold  SaturateOnIntegerOverflow=off  InputSameDT=off
  Unit Delay : UnitDelay  SampleTime=-1  HasFrameUpgradeWarning=on
  Out1 : Outport
  Out2 : Outport  Port=2
  wires:
  Gain3/1 -> Rem/1
  "Low-Pass Filter "/1 -> Out2/1, Scope/1
  Switch2/1 -> Switch/1
  Gain/1 -> Switch2/3
  Gain1/1 -> Switch2/1
  Data Type Conversion/1 -> Gain1/1, Gain/1
  Constant4/1 -> Switch/3
  Gain2/1 -> Gain3/1, Discrete Derivative/1, Scope/2
  Constant3/1 -> Rem/2
  Data Type Conversion1/1 -> Switch2/2
  Constant2/1 -> Data Type Conversion/1
  Switch/1 -> Add1/1, Scope/3
  Discrete Derivative/1 -> "Low-Pass Filter "/1
  Input/1 -> Detect Rise Positive/1
  Input1/1 -> Data Type Conversion1/1
  Detect Rise Positive/1 -> Switch/2
  Rem/1 -> Out1/1
  Unit Delay/1 -> Add1/2
  Add1/1 -> Gain2/1, Unit Delay/1

== system foc_7/Subsystem3/Decoupling ==
  Vq_coupled : Inport
  Vd_coupled : Inport  Port=2
  Add : Sum  Inputs=+++
  Add1 : Sum  Inputs=+-
  Constant1 : Constant  Value=lambda
  Constant2 : Constant  Value=L
  Constant3 : Constant  Value=L
  Product : Product
  Product1 : Product  Inputs=3
  Product2 : Product  Inputs=3
  Vq* : Outport
  Vd* : Outport  Port=2
  wires:
  [W_act] -> Product1/1
  Product/1 -> Add/1
  Product1/1 -> Add/2
  [W_act] -> Product2/1
  Product2/1 -> Add1/2
  Constant3/1 -> Product2/3
  Constant2/1 -> Product1/3
  Constant1/1 -> Product/2
  [Id] -> Product2/2
  [W_act] -> Product/1
  [Iq] -> Product1/2
  Vd_coupled/1 -> Add1/1
  Add1/1 -> Vd*/1  "Vd"
  Add/1 -> Vq*/1  "Vq"
  Vq_coupled/1 -> Add/3

== system foc_7/Subsystem3/PI_Controller_speed ==
  speed_error : Inport
  Abs : Abs  SaturateOnIntegerOverflow=off
  Add : Sum
  Add1 : Sum  Inputs=+-
  Compare To Constant1 : simulink/Logic and Bit Operations/Compare To Constant  relop=<=  const=1e-4  OutDataTypeStr=boolean
  Gain3 : Gain  Gain=Kp_s
  Gain4 : Gain  Gain=Ki_s
  Integrator (Discrete or Continuous) : eeGeneralControl/Integrator (Discrete or Continuous)  LabelModeActiveChoice=Discrete  ExternalReset=level  LimitType=Anti-windup  B=4  A=-inf  Ts=-1
  Product : Product
  Saturation : Saturate  UpperLimit=3.8  LowerLimit=-3.8
  req_Torq : Outport
  wires:
  Saturation/1 -> Add1/2, req_Torq/1
  Add/1 -> Add1/1, Saturation/1
  Gain3/1 -> Add/1
  Integrator (Discrete or Continuous)/1 -> Add/2
  Gain4/1 -> Product/1
  Add1/1 -> Abs/1
  Abs/1 -> Compare To Constant1/1
  speed_error/1 -> Gain3/1, Gain4/1
  Product/1 -> Integrator (Discrete or Continuous)/1
  Compare To Constant1/1 -> Product/2

== system foc_7/Subsystem3/SVPWM ==
  Va : Inport
  Vb : Inport  Port=2
  Vc : Inport  Port=3
  ABC to alpha-beta : Subsystem
  Goto6 : Goto  TagVisibility=global
  PWM : Subsystem
  Repeating Sequence Interpolated1 : simulink/Sources/Repeating Sequence Interpolated  OutValues="[ 0 1/15000  1e-6  ]"  TimeValues=[ 0 1/40000 1/20001]  LookUpMeth=Interpolation-Use End Values  tsamp=1e-6  OutMin=[]  OutMax=[]  OutDataTypeStr=double  OutputDataTypeScalingMode=double  OutDataType=fixdt(0,8)  OutScaling=2^-10
  Scope : Scope  NumInputPorts=3
  Scope1 : Scope  NumInputPorts=3
  Scope2 : Scope  NumInputPorts=3
  Sector selection : Subsystem
  Subsystem3 : Subsystem
  Time equations to Referance signal : Subsystem
  polar form : Subsystem
  time equations : Subsystem
  T1 : Outport
  T3 : Outport  Port=2
  T5 : Outport  Port=3
  tag scope: case1=global, case2=global, case3=global, case4=global
  wires:
  Vb/1 -> ABC to alpha-beta/2(In2)
  time equations/1(T1) -> Scope1/1, Subsystem3/1(In1)
  Va/1 -> ABC to alpha-beta/1(In1)
  Time equations to Referance signal/1(ref1) -> PWM/1(ref1)
  Time equations to Referance signal/2("ref2 ") -> PWM/2(ref2)
  Time equations to Referance signal/3(ref3) -> PWM/3(ref3)
  Vc/1 -> ABC to alpha-beta/3(In3)
  ABC to alpha-beta/1(alpha) -> polar form/1(In1)
  ABC to alpha-beta/2(beta) -> polar form/2(In2)
  PWM/1(PWM1) -> T1/1, Scope2/1
  PWM/2(PWM3) -> T3/1, Scope2/2
  PWM/3(PWM5) -> T5/1, Scope2/3
  polar form/2(Angle) -> Sector selection/1(In1), time equations/3(Angle), Scope/3
  polar form/1(Vr) -> Scope/1, time equations/1(Vref)
  Sector selection/1(K) -> Scope/2, time equations/2(Sector), Goto6/1
  Subsystem3/2(S3) -> [case2]
  Subsystem3/1(S1) -> [case1]
  time equations/3(T0) -> Subsystem3/3(In3), Scope1/3
  time equations/2(T2) -> Scope1/2, Subsystem3/2(In2)
  Subsystem3/4(S5) -> [case4]
  Subsystem3/3(S6) -> [case3]
  Repeating Sequence Interpolated1/1 -> PWM/4(Carrier)

== system foc_7/Subsystem3/Subsystem2 ==
  Iq_error : Inport
  Id_error1 : Inport  Port=2
  PI_Controller_Id : Subsystem
  PI_Controller_Iq : Subsystem
  Vq_coupled : Outport
  Vd_coupled1 : Outport  Port=2
  wires:
  PI_Controller_Id/1(Vd_coupled) -> Vd_coupled1/1
  Id_error1/1 -> PI_Controller_Id/1(Id_error)
  Iq_error/1 -> PI_Controller_Iq/1(Iq_error)
  PI_Controller_Iq/1(Vq_coupled) -> Vq_coupled/1

== system foc_7/Subsystem3/Subsystem3 ==
  Vq : Inport
  Vd : Inport  Port=2
  In2 : Inport  Port=3
  Add : Sum
  Add1 : Sum  Inputs=-+
  Add2 : Sum  Inputs=--
  Add3 : Sum  Inputs=+-
  Cosine : Trigonometry  Operator=cos
  Cosine1 : Trigonometry
  Gain : Gain  Gain=sqrt(3)
  Gain1 : Gain  Gain=1/2
  Gain2 : Gain  Gain=1/2
  Product{,1..3} (4 alike) : Product
  Sin : Trigonometry
  Sin1 : Trigonometry  Operator=cos
  Va : Outport
  Vb : Outport  Port=2
  Vc : Outport  Port=3
  wires:
  Add/1 -> Add3/2, Add2/2, Va/1  "V_beta"
  Product2/1 -> Add1/2
  Product3/1 -> Add1/1
  Cosine/1 -> Product/1
  Sin1/1 -> Product2/1
  Sin/1 -> Product1/1
  Product/1 -> Add/2
  Vd/1 -> Product1/2, Product2/2
  In2/1 -> Sin/1, Cosine/1, Cosine1/1, Sin1/1
  Product1/1 -> Add/1
  Cosine1/1 -> Product3/2
  Add1/1 -> Gain/1  "V_alpha"
  Vq/1 -> Product3/1, Product/2
  Gain1/1 -> Vc/1  "Vc"
  Add3/1 -> Gain2/1
  Gain/1 -> Add2/1, Add3/1
  Add2/1 -> Gain1/1
  Gain2/1 -> Vb/1  "Vb"

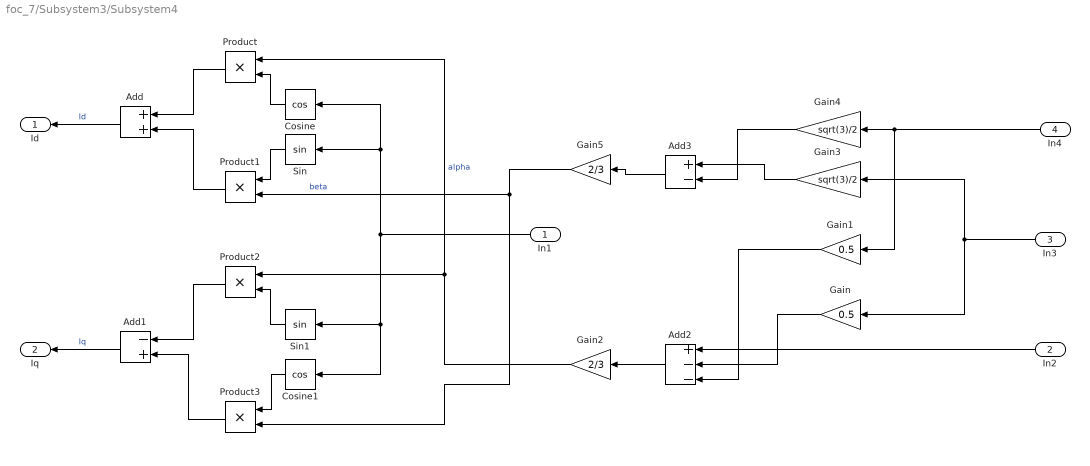
== system foc_7/Subsystem3/Subsystem4 ==
  In1 : Inport
  In2 : Inport  Port=2
  In3 : Inport  Port=3
  In4 : Inport  Port=4
  Add : Sum
  Add1 : Sum  Inputs=-+
  Add2 : Sum  Inputs=+--
  Add3 : Sum  Inputs=+-
  Cosine : Trigonometry  Operator=cos
  Cosine1 : Trigonometry  Operator=cos
  Gain : Gain  Gain=0.5
  Gain1 : Gain  Gain=0.5
  Gain2 : Gain  Gain=2/3
  Gain3 : Gain  Gain=sqrt(3)/2
  Gain4 : Gain  Gain=sqrt(3)/2
  Gain5 : Gain  Gain=2/3
  Product{,1..3} (4 alike) : Product
  Sin : Trigonometry
  Sin1 : Trigonometry
  Id : Outport
  Iq : Outport  Port=2
  wires:
  Add1/1 -> Iq/1  "Iq"
  Add/1 -> Id/1  "Id"
  Product3/1 -> Add1/2
  Product1/1 -> Add/2
  Sin1/1 -> Product2/2
  Sin/1 -> Product1/1
  Product/1 -> Add/1
  Cosine1/1 -> Product3/1
  In1/1 -> Cosine/1, Sin/1, Cosine1/1, Sin1/1
  Product2/1 -> Add1/1
  Cosine/1 -> Product/2
  Gain5/1 -> Product3/2, Product1/2  "beta"
  Gain2/1 -> Product/1, Product2/1  "alpha"
  Add2/1 -> Gain2/1
  In2/1 -> Add2/1
  Gain/1 -> Add2/2
  In4/1 -> Gain1/1, Gain4/1
  Gain1/1 -> Add2/3
  Add3/1 -> Gain5/1
  Gain4/1 -> Add3/2
  In3/1 -> Gain/1, Gain3/1
  Gain3/1 -> Add3/1

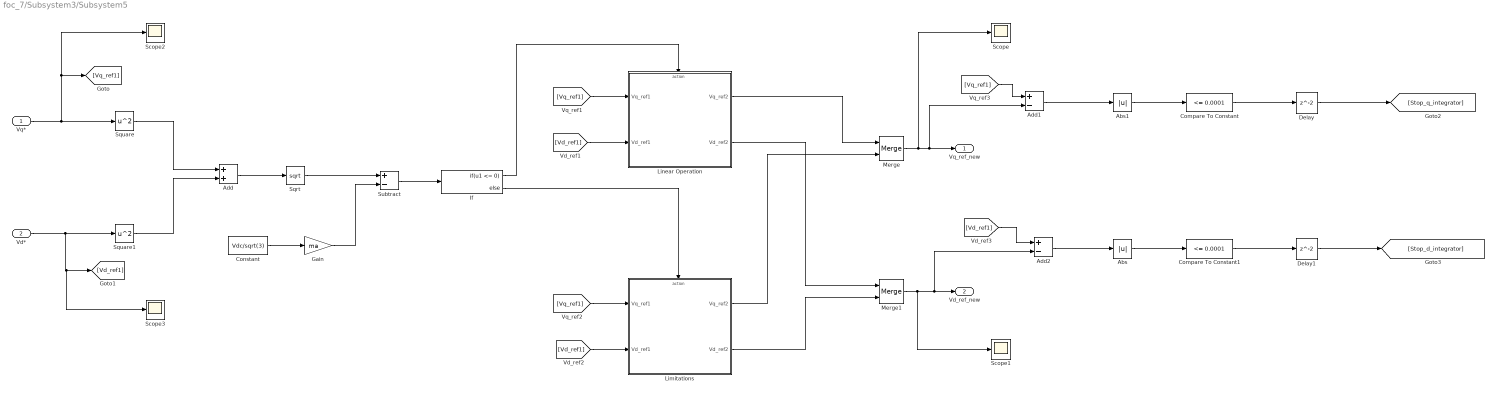
== system foc_7/Subsystem3/Subsystem5 ==
  Vq* : Inport
  Vd* : Inport  Port=2
  Abs : Abs  SaturateOnIntegerOverflow=off
  Abs1 : Abs  SaturateOnIntegerOverflow=off
  Add : Sum
  Add1 : Sum  Inputs=+-
  Add2 : Sum  Inputs=+-
  Compare To Constant : simulink/Logic and Bit Operations/Compare To Constant  relop=<=  const=0.0001  OutDataTypeStr=boolean
  Compare To Constant1 : simulink/Logic and Bit Operations/Compare To Constant  relop=<=  const=0.0001  OutDataTypeStr=boolean
  Constant : Constant  Value=Vdc/sqrt(3)
  Delay : Delay
  Delay1 : Delay
  Gain : Gain  Gain=ma
  If : If  IfExpression=u1 <= 0
  Limitations : Subsystem  TreatAsAtomicUnit=on
  "Linear Operation " : Subsystem  TreatAsAtomicUnit=on
  Merge : Merge
  Merge1 : Merge
  Scope{,1..3} (4 alike) : Scope
  Sqrt : Sqrt
  Square : Math  Operator=square  SignedPower=on
  Square1 : Math  Operator=square  SignedPower=on
  Subtract : Sum  Inputs=+-
  Vq_ref_new : Outport
  Vd_ref_new : Outport  Port=2
  wires:
  Vd*/1 -> Scope3/1, [Vd_ref1], Square1/1
  Vq*/1 -> Scope2/1, [Vq_ref1], Square/1
  Square/1 -> Add/1
  Square1/1 -> Add/2
  Add/1 -> Sqrt/1
  Constant/1 -> Gain/1
  Sqrt/1 -> Subtract/1
  Gain/1 -> Subtract/2
  Subtract/1 -> If/1
  [Vq_ref1] -> "Linear Operation "/1(Vq_ref1)
  [Vd_ref1] -> "Linear Operation "/2(Vd_ref1)
  If/1 -> "Linear Operation "/Action
  If/2 -> Limitations/Action
  [Vq_ref1] -> Limitations/1(Vq_ref1)
  [Vd_ref1] -> Limitations/2(Vd_ref1)
  Limitations/2(Vd_ref2) -> Merge1/2
  "Linear Operation "/2(Vd_ref2) -> Merge1/1
  Limitations/1(Vq_ref2) -> Merge/2
  "Linear Operation "/1(Vq_ref2) -> Merge/1
  Merge/1 -> Scope/1, Add1/2, Vq_ref_new/1
  Merge1/1 -> Scope1/1, Add2/2, Vd_ref_new/1
  [Vq_ref1] -> Add1/1
  [Vd_ref1] -> Add2/1
  Add2/1 -> Abs/1
  Add1/1 -> Abs1/1
  Abs1/1 -> Compare To Constant/1
  Abs/1 -> Compare To Constant1/1
  Compare To Constant/1 -> Delay/1
  Compare To Constant1/1 -> Delay1/1
  Delay/1 -> [Stop_q_integrator]
  Delay1/1 -> [Stop_d_integrator]

== system foc_7/Subsystem3/encoder demux1 ==
  Input : Inport
  Input1 : Inport  Port=2
  Add1 : Sum
  Constant2 : Constant
  Constant3 : Constant  Value=2*pi
  Constant4 : Constant  Value=0
  Data Type Conversion : DataTypeConversion  SaturateOnIntegerOverflow=off  RndMeth=Floor
  Data Type Conversion1 : DataTypeConversion  SaturateOnIntegerOverflow=off  RndMeth=Floor
  Detect Rise Positive : simulink/Logic and Bit Operations/Detect Rise Positive  vinit=0  OutDataTypeStr=uint8
  Discrete Derivative : simulink/Discrete/Discrete Derivative  gainval=1.0  ICPrevScaledInput=0.0  OutMin=[]  OutMax=[]  OutDataType=fixdt(1, 16)  OutScaling=2^-10  DoSatur=off
  Gain : Gain
  Gain1 : Gain  Gain=-1
  Gain2 : Gain  Gain=2*pi /2000
  Gain3 : Gain  Gain=4
  "Low-Pass Filter " : eeGeneralControl/Low-Pass Filter (Discrete or Continuous)  K=1  T=1/100  B=inf  A=-inf  init_option=Inherited from block input  x0=0  Ts=-1
  Rem : Math  Operator=rem
  Scope : Scope  NumInputPorts=3
  Switch : Switch  Criteria=u2 > Threshold  SaturateOnIntegerOverflow=off  InputSameDT=off
  Switch2 : Switch  Criteria=u2 > Threshold  SaturateOnIntegerOverflow=off  InputSameDT=off
  Unit Delay : UnitDelay  SampleTime=-1  HasFrameUpgradeWarning=on
  Out1 : Outport
  Out2 : Outport  Port=2
  wires:
  Gain3/1 -> Rem/1
  "Low-Pass Filter "/1 -> Out2/1, Scope/1
  Switch2/1 -> Switch/1
  Gain/1 -> Switch2/3
  Gain1/1 -> Switch2/1
  Data Type Conversion/1 -> Gain1/1, Gain/1
  Constant4/1 -> Switch/3
  Gain2/1 -> Gain3/1, Discrete Derivative/1, Scope/2
  Constant3/1 -> Rem/2
  Data Type Conversion1/1 -> Switch2/2
  Constant2/1 -> Data Type Conversion/1
  Switch/1 -> Add1/1, Scope/3
  Discrete Derivative/1 -> "Low-Pass Filter "/1
  Input/1 -> Detect Rise Positive/1
  Input1/1 -> Data Type Conversion1/1
  Detect Rise Positive/1 -> Switch/2
  Rem/1 -> Out1/1
  Unit Delay/1 -> Add1/2
  Add1/1 -> Gain2/1, Unit Delay/1

== system foc_7/Subsystem2/SVPWM/ABC to alpha-beta ==
  In1 : Inport
  In2 : Inport  Port=2
  In3 : Inport  Port=3
  Add : Sum  Inputs=+--
  Add1 : Sum  Inputs=+-
  Gain : Gain  Gain=0.5
  Gain1 : Gain  Gain=0.5
  Gain2 : Gain  Gain=2/3
  Gain3 : Gain  Gain=sqrt(3)/2
  Gain4 : Gain  Gain=sqrt(3)/2
  Gain5 : Gain  Gain=2/3
  Scope1 : Scope  NumInputPorts=3
  alpha : Outport
  beta : Outport  Port=2
  wires:
  Gain3/1 -> Add1/1
  In2/1 -> Gain3/1, Scope1/2, Gain/1
  Gain4/1 -> Add1/2
  Add1/1 -> Gain5/1
  Gain1/1 -> Add/3
  In3/1 -> Scope1/3, Gain4/1, Gain1/1
  Gain/1 -> Add/2
  In1/1 -> Add/1, Scope1/1
  Add/1 -> Gain2/1
  Gain2/1 -> alpha/1  "alpha"
  Gain5/1 -> beta/1  "beta"

== system foc_7/Subsystem2/SVPWM/PWM ==
  ref1 : Inport
  ref2 : Inport  Port=2
  ref3 : Inport  Port=3
  Carrier : Inport  Port=4
  Relational Operator : RelationalOperator  OutDataTypeStr=boolean  RndMeth=Simplest  InputSameDT=off
  Relational Operator1 : RelationalOperator  OutDataTypeStr=boolean  RndMeth=Simplest  InputSameDT=off
  Relational Operator2 : RelationalOperator  OutDataTypeStr=boolean  RndMeth=Simplest  InputSameDT=off
  PWM1 : Outport
  PWM3 : Outport  Port=2
  PWM5 : Outport  Port=3
  wires:
  ref1/1 -> Relational Operator/1
  ref2/1 -> Relational Operator1/1
  ref3/1 -> Relational Operator2/1
  Carrier/1 -> Relational Operator/2, Relational Operator2/2, Relational Operator1/2
  Relational Operator/1 -> PWM1/1
  Relational Operator1/1 -> PWM3/1
  Relational Operator2/1 -> PWM5/1

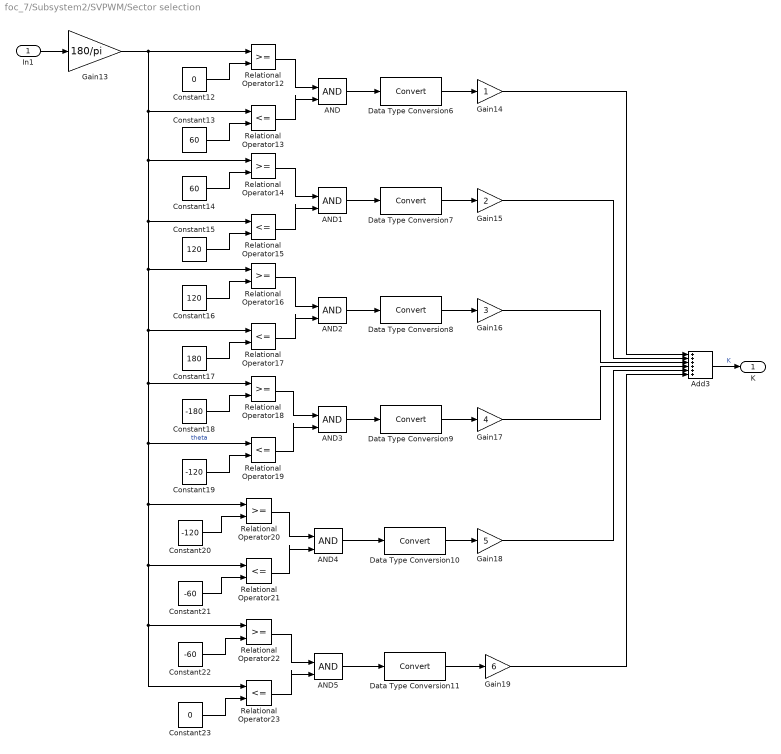
== system foc_7/Subsystem2/SVPWM/Sector selection ==
  In1 : Inport
  AND{,1..5} (6 alike) : Logic  IconShape=distinctive  AllPortsSameDT=off  OutDataTypeStr=boolean
  Add3 : Sum  Inputs=++++++
  Constant12 : Constant  Value=0
  Constant13 : Constant  Value=60
  Constant14 : Constant  Value=60
  Constant15 : Constant  Value=120
  Constant16 : Constant  Value=120
  Constant17 : Constant  Value=180
  Constant18 : Constant  Value=-180
  Constant19 : Constant  Value=-120
  Constant20 : Constant  Value=-120
  Constant21 : Constant  Value=-60
  Constant22 : Constant  Value=-60
  Constant23 : Constant  Value=0
  Data Type Conversion{6..11} (6 alike) : DataTypeConversion  SaturateOnIntegerOverflow=off  RndMeth=Floor
  Gain13 : Gain  Gain=180/pi
  Gain14 : Gain
  Gain15 : Gain  Gain=2
  Gain16 : Gain  Gain=3
  Gain17 : Gain  Gain=4
  Gain18 : Gain  Gain=5
  Gain19 : Gain  Gain=6
  Relational Operator{12,14,16,18,20,22} (6 alike) : RelationalOperator  OutDataTypeStr=boolean  RndMeth=Simplest  InputSameDT=off
  Relational Operator{13,15,17,19,21,23} (6 alike) : RelationalOperator  Operator=<=  OutDataTypeStr=boolean  RndMeth=Simplest  InputSameDT=off
  K : Outport
  wires:
  AND2/1 -> Data Type Conversion8/1
  Relational Operator14/1 -> AND1/1
  Relational Operator12/1 -> AND/1
  Data Type Conversion10/1 -> Gain18/1
  Data Type Conversion8/1 -> Gain16/1
  Relational Operator19/1 -> AND3/2
  Gain13/1 -> Relational Operator14/1, Relational Operator18/1, Relational Operator19/1, Relational Operator20/1, Relational Operator22/1, Relational Operator23/1, Relational Operator21/1, Relational Operator17/1, Relational Operator16/1, Relational Operator15/1, Relational Operator13/1, Relational Operator12/1  "theta"
  Data Type Conversion6/1 -> Gain14/1
  Constant21/1 -> Relational Operator21/2
  Constant19/1 -> Relational Operator19/2
  Gain19/1 -> Add3/6
  Constant18/1 -> Relational Operator18/2
  AND4/1 -> Data Type Conversion10/1
  Constant22/1 -> Relational Operator22/2
  Relational Operator22/1 -> AND5/1
  Relational Operator18/1 -> AND3/1
  Gain15/1 -> Add3/2
  Relational Operator23/1 -> AND5/2
  Data Type Conversion11/1 -> Gain19/1
  Constant16/1 -> Relational Operator16/2
  Data Type Conversion7/1 -> Gain15/1
  Constant23/1 -> Relational Operator23/2
  Relational Operator20/1 -> AND4/1
  Gain18/1 -> Add3/5
  Gain14/1 -> Add3/1
  AND1/1 -> Data Type Conversion7/1
  Constant14/1 -> Relational Operator14/2
  Relational Operator16/1 -> AND2/1
  Relational Operator17/1 -> AND2/2
  Gain17/1 -> Add3/4
  Constant12/1 -> Relational Operator12/2
  Gain16/1 -> Add3/3
  Relational Operator13/1 -> AND/2
  Relational Operator15/1 -> AND1/2
  Data Type Conversion9/1 -> Gain17/1
  AND/1 -> Data Type Conversion6/1
  Constant13/1 -> Relational Operator13/2
  Relational Operator21/1 -> AND4/2
  AND3/1 -> Data Type Conversion9/1
  Constant20/1 -> Relational Operator20/2
  Constant17/1 -> Relational Operator17/2
  AND5/1 -> Data Type Conversion11/1
  Constant15/1 -> Relational Operator15/2
  Add3/1 -> K/1  "K"
  In1/1 -> Gain13/1

== system foc_7/Subsystem2/SVPWM/Subsystem3 ==
  In1 : Inport
  In2 : Inport  Port=2
  In3 : Inport  Port=3
  Add10 : Sum
  Add8 : Sum  Inputs=+++
  Add9 : Sum
  Gain{9..12} (4 alike) : Gain  Gain=0.5
  S1 : Outport
  S3 : Outport  Port=2
  S6 : Outport  Port=3
  S5 : Outport  Port=4
  wires:
  In3/1 -> Gain9/1, Gain10/1, Gain12/1, Gain11/1
  Gain11/1 -> Add10/2
  Gain9/1 -> Add8/3
  Gain10/1 -> Add9/2
  Add8/1 -> S1/1  "S1"
  In2/1 -> Add9/1, Add8/2
  In1/1 -> Add10/1, Add8/1
  Add9/1 -> S3/1  "S3"
  Gain12/1 -> S5/1  "S5"
  Add10/1 -> S6/1  "S6"

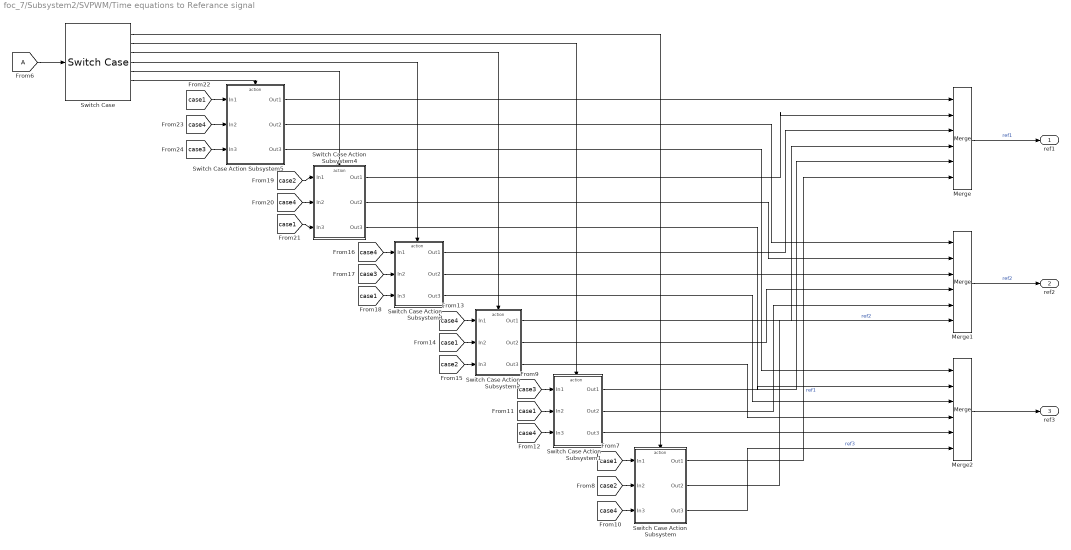
== system foc_7/Subsystem2/SVPWM/Time equations to Referance signal ==
  From6 : From  TagVisibility=global
  Merge : Merge  Inputs=6
  Merge1 : Merge  Inputs=6
  Merge2 : Merge  Inputs=6
  Switch Case : SwitchCase  CaseConditions={1 2 3 4 5 6}
  Switch Case Action Subsystem : Subsystem  TreatAsAtomicUnit=on
  Switch Case Action Subsystem1 : Subsystem  TreatAsAtomicUnit=on
  Switch Case Action Subsystem2 : Subsystem  TreatAsAtomicUnit=on
  Switch Case Action Subsystem3 : Subsystem  TreatAsAtomicUnit=on
  Switch Case Action Subsystem4 : Subsystem  TreatAsAtomicUnit=on
  Switch Case Action Subsystem5 : Subsystem  TreatAsAtomicUnit=on
  ref1 : Outport
  "ref2 " : Outport  Port=2
  ref3 : Outport  Port=3
  wires:
  [case3] -> Switch Case Action Subsystem5/3(In3)
  Switch Case Action Subsystem4/1(Out1) -> Merge/2
  [case1] -> Switch Case Action Subsystem2/2(In2)
  Switch Case Action Subsystem3/2(Out2) -> Merge1/3
  [case4] -> Switch Case Action Subsystem3/1(In1)
  Switch Case/4 -> Switch Case Action Subsystem3/Action
  [case2] -> Switch Case Action Subsystem4/1(In1)
  Switch Case/6 -> Switch Case Action Subsystem5/Action
  [case4] -> Switch Case Action Subsystem1/3(In3)
  [case1] -> Switch Case Action Subsystem5/1(In1)
  [case3] -> Switch Case Action Subsystem1/1(In1)
  Merge/1 -> ref1/1  "ref1"
  Switch Case Action Subsystem5/1(Out1) -> Merge/1
  Switch Case/5 -> Switch Case Action Subsystem4/Action
  Switch Case Action Subsystem4/3(Out3) -> Merge2/2
  [case1] -> Switch Case Action Subsystem/1(In1)
  Switch Case Action Subsystem2/3(Out3) -> Merge2/4
  Switch Case Action Subsystem4/2(Out2) -> Merge1/2
  Switch Case/3 -> Switch Case Action Subsystem2/Action
  Switch Case Action Subsystem/2(Out2) -> Merge1/6  "ref2"
  Switch Case Action Subsystem3/3(Out3) -> Merge2/3
  Switch Case Action Subsystem5/2(Out2) -> Merge1/1
  [case3] -> Switch Case Action Subsystem3/2(In2)
  Switch Case/2 -> Switch Case Action Subsystem1/Action
  Switch Case Action Subsystem2/1(Out1) -> Merge/4
  Switch Case Action Subsystem2/2(Out2) -> Merge1/4
  [case1] -> Switch Case Action Subsystem4/3(In3)
  [case4] -> Switch Case Action Subsystem5/2(In2)
  Switch Case/1 -> Switch Case Action Subsystem/Action
  Switch Case Action Subsystem5/3(Out3) -> Merge2/1
  [case4] -> Switch Case Action Subsystem2/1(In1)
  Switch Case Action Subsystem3/1(Out1) -> Merge/3
  [case4] -> Switch Case Action Subsystem/3(In3)
  Merge2/1 -> ref3/1
  From6/1 -> Switch Case/1
  [case4] -> Switch Case Action Subsystem4/2(In2)
  [case2] -> Switch Case Action Subsystem/2(In2)
  [case2] -> Switch Case Action Subsystem2/3(In3)
  [case1] -> Switch Case Action Subsystem3/3(In3)
  Switch Case Action Subsystem1/2(Out2) -> Merge1/5
  Switch Case Action Subsystem/1(Out1) -> Merge/6  "ref1"
  Switch Case Action Subsystem1/1(Out1) -> Merge/5
  Switch Case Action Subsystem/3(Out3) -> Merge2/6  "ref3"
  Switch Case Action Subsystem1/3(Out3) -> Merge2/5
  [case1] -> Switch Case Action Subsystem1/2(In2)
  Merge1/1 -> "ref2 "/1  "ref2"

== system foc_7/Subsystem2/SVPWM/polar form ==
  In1 : Inport
  In2 : Inport  Port=2
  Add2 : Sum
  Atan2 : Trigonometry  Operator=atan2
  Math Function : Math  Operator=square  SignedPower=on
  Math Function1 : Math  Operator=square  SignedPower=on
  Saturation2 : Saturate  UpperLimit=0.95 * Vdc /sqrt(3)  LowerLimit=0
  Scope1 : Scope  NumInputPorts=2
  Scope2 : Scope  NumInputPorts=2
  Square Root : Sqrt
  Vr : Outport
  Angle : Outport  Port=2
  wires:
  In2/1 -> Scope2/2, Atan2/2, Math Function1/1
  In1/1 -> Scope2/1, Atan2/1, Math Function/1
  Math Function1/1 -> Add2/2
  Add2/1 -> Square Root/1
  Math Function/1 -> Add2/1
  Atan2/1 -> Angle/1
  Square Root/1 -> Saturation2/1, Scope1/1  "Vr"
  Saturation2/1 -> Vr/1, Scope1/2

== system foc_7/Subsystem2/SVPWM/time equations ==
  Vref : Inport
  Sector : Inport  Port=2
  Angle : Inport  Port=3
  Add4 : Sum  Inputs=+-
  Add5 : Sum  Inputs=+-
  Add6 : Sum  Inputs=+-
  Add7 : Sum  Inputs=+--
  Constant : Constant  Value=T_period
  Divide : Product  Inputs=*/
  Gain6 : Gain  Gain=sqrt(3)*(T_period)
  Gain7 : Gain  Gain=pi/3
  Gain8 : Gain  Gain=pi/3
  Product : Product
  Product1 : Product
  Sin1 : Trigonometry
  Sin4 : Trigonometry
  Vdc : Constant  Value=Vdc
  const : Constant
  T1 : Outport
  T2 : Outport  Port=2
  T0 : Outport  Port=3
  wires:
  Vdc/1 -> Divide/2
  Gain6/1 -> Product1/1, Product/1
  Divide/1 -> Gain6/1
  Add6/1 -> Gain8/1
  Constant/1 -> Add7/1
  Gain7/1 -> Add4/1
  Add5/1 -> Sin4/1
  Sin4/1 -> Product1/2
  Sin1/1 -> Product/2
  Gain8/1 -> Add5/2
  Angle/1 -> Add5/1, Add4/2
  const/1 -> Add6/2
  Product1/1 -> T2/1, Add7/3  "T2"
  Sector/1 -> Gain7/1, Add6/1
  Add4/1 -> Sin1/1
  Vref/1 -> Divide/1
  Product/1 -> Add7/2, T1/1  "T1"
  Add7/1 -> T0/1

== system foc_7/Subsystem2/Subsystem2/PI_Controller_Id ==
  Id_error : Inport
  Discrete-Time Integrator1 : DiscreteIntegrator  SampleTime=-1  ICPrevOutput=DiscIntNeverNeededParam  ICPrevScaledInput=DiscIntNeverNeededParam
  Gain1 : Gain  Gain=Kp
  Gain2 : Gain  Gain=Ki
  Product : Product
  Scope : Scope  NumInputPorts=2
  Scope1 : Scope
  Sum1 : Sum
  Vd_coupled : Outport
  wires:
  [Stop_d_integrator] -> Scope/2, Product/1
  Sum1/1 -> Scope1/1, Vd_coupled/1
  Product/1 -> Scope/1, Discrete-Time Integrator1/1
  Gain2/1 -> Product/2
  Discrete-Time Integrator1/1 -> Sum1/2
  Gain1/1 -> Sum1/1
  Id_error/1 -> Gain2/1, Gain1/1

== system foc_7/Subsystem2/Subsystem2/PI_Controller_Iq ==
  Iq_error : Inport
  Discrete-Time Integrator1 : DiscreteIntegrator  SampleTime=-1  ICPrevOutput=DiscIntNeverNeededParam  ICPrevScaledInput=DiscIntNeverNeededParam
  Gain1 : Gain  Gain=Kp
  Gain2 : Gain  Gain=Ki
  Product : Product
  Scope : Scope  NumInputPorts=2
  Scope1 : Scope
  Sum1 : Sum
  Vq_coupled : Outport
  wires:
  Product/1 -> Scope/1, Discrete-Time Integrator1/1
  Iq_error/1 -> Gain2/1, Gain1/1
  Discrete-Time Integrator1/1 -> Sum1/2
  Gain1/1 -> Sum1/1
  Gain2/1 -> Product/2
  [Stop_q_integrator] -> Scope/2, Product/1
  Sum1/1 -> Scope1/1, Vq_coupled/1
